simulink model "AUV_ControlsPreliminary"  (R2020b)
settings: Solver=ode23t  StartTime=0.0  StopTime=300  MaxStep=0.01  RelTol=1e-3  EnableMultiTasking=on
PreLoadFcn:
  | AUV_VehicleParameters;
  | Vehicle.Body.markeropacity = 0;
model workspace: external: MATLAB File AUV_DataFile_ORIG.m (data not in the file)
undefined symbols (not defined in the file or in its folder): Environment, Multibody, Newton, Raphson, smiData, X, x, Y, y, Z
libraries: sm_lib x3123, nesl_utility x51, sharedutil x8, pid_lib x6, AUVCustomPrimitives_Lib x4, shared6dof x1, aerolibasang x1, aerolibadyn x1, SignalEditorBlockLib x1
(part 4 of 62)

== system AUV_ControlsPreliminary/AUV/Muiltibody/World/Sea Floor ==
  T1 : sm_lib/Frames and Transforms/Rigid Transform  TranslationMethod=Cartesian  TranslationStandardOffset=0  TranslationLengthUnit=m  TranslationStandardAxis=+Z  TranslationCartesianOffset=[-Environment.seafloortileside 0 Environment.seafloordepth]  TranslationROffset=0  TranslationROffsetUnits=m  TranslationZOffset=0  TranslationZOffsetUnits=m  TranslationThetaOffset=0  TranslationThetaOffsetUnits=deg  RotationMethod=None  RotationAngleUnits=deg  RotationStandardAxis=+Z  RotationAngle=0.0  RotationArbitraryAxis=[0 0 1]  FollAlignAxisA=+X  BaseAlignAxisA=+Y  FollAlignAxisB=+Y  BaseAlignAxisB=+Z  RotationSequenceAxes=FollowerAxes  RotationSequence=XYX  RotationSequenceAngles=[0 0 0]  RotationSequenceAnglesUnits=deg  RotationMatrix=[1 0 0; 0 1 0; 0 0 1]
  Tiled Grid : Subsystem  mask(Tiled Grid){side=Environment.seafloortileside, thick=0.004, color1=[0 0.8 0.4], color2=[0 0.6 0.8], opacity=Environment.seaflooropacity}
      mask prompts: side "Tile Side (m) :"; thick "Tile Thickness (m) :"; color1 "First Color [RGB] :"; color2 "Second Color [RGB] :"; opacity "Tile Opacity (0...1) :"
      mask help: This block creates a tiled grid composed of square tiles.
  W : PMIOPort  Side=Left
  connections:
  W/RConn1 -- T1/LConn1
  T1/RConn1 -- Tiled Grid/LConn1

== system AUV_ControlsPreliminary/AUV/Singlebody/AUV Mechanics/DCMbe to R ==
  DCMbe : Inport
  Transpose : Math  Operator=transpose  SaturateOnIntegerOverflow=on
  R : Outport
  wires:
  Transpose/1 -> R/1
  DCMbe/1 -> Transpose/1

== system AUV_ControlsPreliminary/AUV/Singlebody/AUV Mechanics/Incidence Angles ==
  Vb : Inport
  "Incidence, Sideslip & Speed" : Subsystem
      mask Display:
      | port_label('input',1,'V_b','texmode','on');
      | port_label('output',1,'\alpha','texmode','on');
      | port_label('output',2,'\beta','texmode','on');
      | port_label('output',3,'V','texmode','on');
  alpha : Outport  Unit=rad
  beta : Outport  Port=2  Unit=rad
  V : Outport  Port=3  Unit=m/s
  wires:
  Vb/1 -> "Incidence, Sideslip & Speed"/1(Vb)
  "Incidence, Sideslip & Speed"/1(Alpha) -> alpha/1
  "Incidence, Sideslip & Speed"/3(V) -> V/1
  "Incidence, Sideslip & Speed"/2(Beta) -> beta/1

== system AUV_ControlsPreliminary/AUV/Singlebody/Hydro Forces & Moments/Added Mass Forces ==
  note: NOTE:
      | All added mass forces are already calculated with respect to the vehicle CoM
  AMFxyz : Inport
  AMMxyz : Inport  Port=2
  AMCFxyz : Inport  Port=3
  AMCMxyz : Inport  Port=4
  Sum : Sum  Inputs=|++
  Sum1 : Sum  Inputs=|++
  Fxyz : Outport
  Mxyz : Outport  Port=2
  wires:
  AMFxyz/1 -> Sum/1
  Sum/1 -> Fxyz/1
  AMCFxyz/1 -> Sum/2
  AMMxyz/1 -> Sum1/1
  Sum1/1 -> Mxyz/1
  AMCMxyz/1 -> Sum1/2

== system AUV_ControlsPreliminary/AUV/Singlebody/Hydro Forces & Moments/Hydrostatic Forces ==
  note: NOTE:
      | Both, the gravitaional force and the buoyancy force need to be transformed from inertial frame coordinates to body frame coordinates.
      | Additionally, the buoyancy force needs to be translated from the CoB to the CoM and we need to account for the corresponding moment.
  DCM : Inport
  Bz : Inport  Port=2
  Wz : Inport  Port=3
  CoB Moment Arm : Constant  Value=Vehicle.Body.Full.BArm
  Fb x (CoM-CoB) : sharedutil/3x3 Cross Product  aMode=aMode
      settings: SourceProductBaseCode=AE,PW,MT,UV,VE,VP
  Inertial to Body Buoyancy : Product  Multiplication=Matrix(*)
  Inertial to Body Weight : Product  Multiplication=Matrix(*)
  Reshape : Reshape  OutputDimensionality=Column vector (2-D)
  Sum : Sum  Inputs=++|
  Vector Concatenate : Concatenate  NumInputs=3
  Vector Concatenate1 : Concatenate  NumInputs=3
  zeroB : Constant  Value=0
  zeroW : Constant  Value=0
  Fxyz : Outport
  Mxyz : Outport  Port=2
  wires:
  Vector Concatenate1/1 -> Inertial to Body Weight/2
  DCM/1 -> Inertial to Body Weight/1, Inertial to Body Buoyancy/1
  Sum/1 -> Fxyz/1
  Inertial to Body Buoyancy/1 -> Sum/1, Fb x (CoM-CoB)/1  "Fb"
  zeroW/1 -> Vector Concatenate1/2, Vector Concatenate1/1
  Vector Concatenate/1 -> Inertial to Body Buoyancy/2
  zeroB/1 -> Vector Concatenate/2, Vector Concatenate/1
  Inertial to Body Weight/1 -> Sum/2  "Fg"
  Bz/1 -> Vector Concatenate/3
  Wz/1 -> Vector Concatenate1/3
  CoB Moment Arm/1 -> Reshape/1
  Fb x (CoM-CoB)/1 -> Mxyz/1
  Reshape/1 -> Fb x (CoM-CoB)/2

== system AUV_ControlsPreliminary/AUV/Singlebody/Hydro Forces & Moments/Lift and Drag Forces ==
  note: NOTE:
      | All lift and drag forces are already calculated with respect to the vehicle CoM
  LDFxyz : Inport
  LDMxyz : Inport  Port=2
  Fxyz : Outport
  Mxyz : Outport  Port=2
  wires:
  LDMxyz/1 -> Mxyz/1
  LDFxyz/1 -> Fxyz/1

== system AUV_ControlsPreliminary/AUV/Singlebody/Propellers & Thrusters/Horizontal Tunnel Thrusters ==
  note: NOTE:
      | Horizontal tunnel thruster vectors actuate in the +Y direction of the body frame
  BHTf : Inport
  SHTf : Inport  Port=2
  BHT Moment Arm wrt to CoM : Constant  Value=[Vehicle.Thruster.BHarmX,0,Vehicle.Thruster.BHarmZ]
  Fbht x (CoM-BHT) : sharedutil/3x3 Cross Product  aMode=aMode
      settings: SourceProductBaseCode=AE,PW,MT,UV,VE,VP
  Fsht x (CoM-SHT) : sharedutil/3x3 Cross Product  aMode=aMode
      settings: SourceProductBaseCode=AE,PW,MT,UV,VE,VP
  Reshape : Reshape  OutputDimensionality=Column vector (2-D)
  Reshape1 : Reshape  OutputDimensionality=Column vector (2-D)
  SHT Moment Arm wrt CoM : Constant  Value=[Vehicle.Thruster.SHarmX,0,Vehicle.Thruster.SHarmZ]
  Sum : Sum  Inputs=|++
  Sum1 : Sum  Inputs=|++
  Vector Concatenate : Concatenate  NumInputs=3
  Vector Concatenate1 : Concatenate  NumInputs=3
  zeroBHTf : Constant  Value=0
  zeroSHTf : Constant  Value=0
  Fxyz : Outport
  Mxyz : Outport  Port=2
  wires:
  zeroSHTf/1 -> Vector Concatenate1/3, Vector Concatenate1/1
  zeroBHTf/1 -> Vector Concatenate/3, Vector Concatenate/1
  Vector Concatenate/1 -> Fbht x (CoM-BHT)/1, Sum/1
  Vector Concatenate1/1 -> Fsht x (CoM-SHT)/1, Sum/2
  Sum/1 -> Fxyz/1
  BHT Moment Arm wrt to CoM/1 -> Reshape/1
  Reshape/1 -> Fbht x (CoM-BHT)/2
  SHT Moment Arm wrt CoM/1 -> Reshape1/1
  Sum1/1 -> Mxyz/1
  Fbht x (CoM-BHT)/1 -> Sum1/1
  Fsht x (CoM-SHT)/1 -> Sum1/2
  Reshape1/1 -> Fsht x (CoM-SHT)/2
  BHTf/1 -> Vector Concatenate/2
  SHTf/1 -> Vector Concatenate1/2

== system AUV_ControlsPreliminary/AUV/Singlebody/Propellers & Thrusters/Main Propellers ==
  note: NOTE:
      | Main propellers thrust vectors actuate in the +X direction of the body frame
  SPf : Inport
  PPf : Inport  Port=2
  Fpp x (CoM-PP) : sharedutil/3x3 Cross Product  aMode=aMode
      settings: SourceProductBaseCode=AE,PW,MT,UV,VE,VP
  Fsp x (CoM-SP) : sharedutil/3x3 Cross Product  aMode=aMode
      settings: SourceProductBaseCode=AE,PW,MT,UV,VE,VP
  PP Moment Arm wrt to CoM : Constant  Value=[0,Vehicle.Prop.PParmY,Vehicle.Prop.PParmZ]
  Reshape : Reshape  OutputDimensionality=Column vector (2-D)
  Reshape1 : Reshape  OutputDimensionality=Column vector (2-D)
  SP Moment Arm wrt to CoM : Constant  Value=[0,Vehicle.Prop.SParmY,Vehicle.Prop.SParmZ]
  Sum : Sum  Inputs=|++
  Sum1 : Sum  Inputs=|++
  Vector Concatenate : Concatenate  NumInputs=3
  Vector Concatenate1 : Concatenate  NumInputs=3
  zeroPPf : Constant  Value=0
  zeroSPf : Constant  Value=0
  Fxyz : Outport
  Mxyz : Outport  Port=2
  wires:
  PPf/1 -> Vector Concatenate1/1
  zeroSPf/1 -> Vector Concatenate/2, Vector Concatenate/3
  zeroPPf/1 -> Vector Concatenate1/2, Vector Concatenate1/3
  Vector Concatenate/1 -> Fsp x (CoM-SP)/1, Sum/1
  Vector Concatenate1/1 -> Fpp x (CoM-PP)/1, Sum/2
  SPf/1 -> Vector Concatenate/1
  Sum/1 -> Fxyz/1
  SP Moment Arm wrt to CoM/1 -> Reshape/1
  Reshape/1 -> Fsp x (CoM-SP)/2
  PP Moment Arm wrt to CoM/1 -> Reshape1/1
  Sum1/1 -> Mxyz/1
  Fsp x (CoM-SP)/1 -> Sum1/1
  Fpp x (CoM-PP)/1 -> Sum1/2
  Reshape1/1 -> Fpp x (CoM-PP)/2

== system AUV_ControlsPreliminary/AUV/Singlebody/Propellers & Thrusters/Vertical Tunnel Thrusters ==
  note: NOTE:
      | Vertical tunnel thruster vectors actuate in the +Z direction of the body frame
  BVTf : Inport
  SVTf : Inport  Port=2
  BVT Moment Arm wrt to CoM : Constant  Value=[Vehicle.Thruster.BVarmX,0,0]
  Fbvt x (CoM-BVT) : sharedutil/3x3 Cross Product  aMode=aMode
      settings: SourceProductBaseCode=AE,PW,MT,UV,VE,VP
  Fsvt x (CoM-SVT) : sharedutil/3x3 Cross Product  aMode=aMode
      settings: SourceProductBaseCode=AE,PW,MT,UV,VE,VP
  Reshape : Reshape  OutputDimensionality=Column vector (2-D)
  Reshape1 : Reshape  OutputDimensionality=Column vector (2-D)
  SVT Moment Arm wrt CoM : Constant  Value=[Vehicle.Thruster.SVarmX,0,0]
  Sum : Sum  Inputs=|++
  Sum1 : Sum  Inputs=|++
  Vector Concatenate : Concatenate  NumInputs=3
  Vector Concatenate1 : Concatenate  NumInputs=3
  zeroBVTf : Constant  Value=0
  zeroSVTf : Constant  Value=0
  Fxyz : Outport
  Mxyz : Outport  Port=2
  wires:
  Reshape1/1 -> Fsvt x (CoM-SVT)/2
  Fsvt x (CoM-SVT)/1 -> Sum1/2
  Fbvt x (CoM-BVT)/1 -> Sum1/1
  Sum1/1 -> Mxyz/1
  SVT Moment Arm wrt CoM/1 -> Reshape1/1
  Reshape/1 -> Fbvt x (CoM-BVT)/2
  BVT Moment Arm wrt to CoM/1 -> Reshape/1
  Sum/1 -> Fxyz/1
  Vector Concatenate1/1 -> Sum/2, Fsvt x (CoM-SVT)/1
  Vector Concatenate/1 -> Sum/1, Fbvt x (CoM-BVT)/1
  BVTf/1 -> Vector Concatenate/3
  zeroBVTf/1 -> Vector Concatenate/2, Vector Concatenate/1
  zeroSVTf/1 -> Vector Concatenate1/2, Vector Concatenate1/1
  SVTf/1 -> Vector Concatenate1/3

== system AUV_ControlsPreliminary/Dive Controls/Thrust Controls/Depth and Pitch Control/Main Propellers Thrust Offset Compensation ==
  PPf : Inport
  SPf : Inport  Port=2
  Bow Vertical Thruster Moment Arm : Constant  Value=-Vehicle.Thruster.BVarmX
  Main Propellers Moment Arm : Constant  Value=-Vehicle.Prop.SParmZ
  Product : Product
  Product1 : Product
  Product2 : Product  Inputs=*/
  Stern Vertical Thruster Moment Arm : Constant  Value=Vehicle.Thruster.SVarmX
  Sum : Sum  Inputs=|++
  Sum1 : Sum  Inputs=|++
  VTf : Outport
  wires:
  Product1/1 -> Sum/1
  Product/1 -> Sum/2
  SPf/1 -> Product/1
  PPf/1 -> Product1/1
  Main Propellers Moment Arm/1 -> Product1/2, Product/2
  Bow Vertical Thruster Moment Arm/1 -> Sum1/1
  Stern Vertical Thruster Moment Arm/1 -> Sum1/2
  Sum/1 -> Product2/1
  Sum1/1 -> Product2/2
  Product2/1 -> VTf/1

== system AUV_ControlsPreliminary/Dive Controls/Thrust Controls/Heading and Yaw Control/psidot ==
  pqr : Inport
  phithetapsi : Inport  Port=2
  Mux1 : Mux  Inputs=[3 3 3]
  psidot : Fcn  Expr=(u[2]*u[4]+u[3]*u[7])/u[8]
  sincos : Trigonometry  Operator=sincos
  psid : Outport  Unit=rad/s  InitialOutput=0  VectorParamsAs1DForOutWhenUnconnected=off
  wires:
  sincos/2 -> Mux1/3
  sincos/1 -> Mux1/2
  phithetapsi/1 -> sincos/1
  pqr/1 -> Mux1/1
  Mux1/1 -> psidot/1
  psidot/1 -> psid/1

== system AUV_ControlsPreliminary/Dive Controls/Thrust Controls/Heading and Yaw Control/side slip compensation ==
  note: NOTE: Lateral force offset is distributed based of the horizontal thrusters moment arms to make the net torque contribution zero
  v : Inport
  BowHTForce : Gain  Gain=Vehicle.Thruster.SHarmX/(-Vehicle.Thruster.BHarmX+Vehicle.Thruster.SHarmX)
  Gain1 : Gain  Gain=-1
  PIv : pid_lib/PID Controller  Controller=PI  Form=Parallel  TimeDomain=Continuous-time  UseExternalTs=off  SampleTime=-1  IntegratorMethod=Forward Euler  FilterMethod=Forward Euler  ControllerParametersSource=internal  P=10  I=0.01  D=0  UseFilter=on  N=100  TunerSelectOption=Transfer Function Based (PID Tuner App)  InitialConditionSource=internal  InitialConditionForIntegrator=0  InitialConditionForFilter=0  DifferentiatorICPrevScaledInput=0  ExternalReset=none  TrackingMode=off  Kt=1  LimitOutput=off  SatLimitsSource=internal  UpperSaturationLimit=inf  LowerSaturationLimit=-inf  LinearizeAsGain=on  AntiWindupMode=none  Kb=1  POutMin=[]  POutMax=[]  IOutMin=[]  IOutMax=[]  DOutMin=[]  DOutMax=[]  NOutMin=[]  NOutMax=[]  SumOutMin=[]  SumOutMax=[]  SaturationOutMin=[]  SaturationOutMax=[]  PParamMin=[]  PParamMax=[]  IParamMin=[]  IParamMax=[]  DParamMin=[]  DParamMax=[]  NParamMin=[]  NParamMax=[]  KbParamMin=[]  KbParamMax=[]  KtParamMin=[]  KtParamMax=[]  KbOutMin=[]  KbOutMax=[]  KtOutMin=[]  KtOutMax=[]  IntegratorOutMin=[]  IntegratorOutMax=[]  FilterOutMin=[]  FilterOutMax=[]  SumI1OutMin=[]  SumI1OutMax=[]  SumI2OutMin=[]  SumI2OutMax=[]  SumI3OutMin=[]  SumI3OutMax=[]  SumI4OutMin=[]  SumI4OutMax=[]  SumDOutMin=[]  SumDOutMax=[]  DifferentiatorOutMin=[]  DifferentiatorOutMax=[]  FilterDiffOutCoefMin=[]  FilterDiffOutCoefMax=[]  ReciprocalOutMin=[]  ReciprocalOutMax=[]  SumDenOutMin=[]  SumDenOutMax=[]  SumNumOutMin=[]  SumNumOutMax=[]  DivideOutMin=[]  DivideOutMax=[]  UdiffTsProdOutMin=[]  UdiffTsProdOutMax=[]  NTsProdOutMin=[]  NTsProdOutMax=[]  UintegralTsProdOutMin=[]  UintegralTsProdOutMax=[]  UngainTsProdOutMin=[]  UngainTsProdOutMax=[]  IntegratorContinuousStateAttributes=''  IntegratorStateMustResolveToSignalObject=off  IntegratorRTWStateStorageClass=Auto  FilterContinuousStateAttributes=''  FilterStateMustResolveToSignalObject=off  FilterRTWStateStorageClass=Auto  ParallelPVariant=InternalParameters  IdealPVariant=Disabled  IVariant=InternalParameters  DVariant=Disabled  IntegratorVariant=Continuous  SatVariant=Disabled  AWVariant=Passthrough  PCopyVariant=Disabled  TRVariant=Disabled  FdbkBlocksVariant=Forward  IdealPFdbkVariant=Disabled  SatFdbkVariant=Disabled  DerivativeFilterVariant=Disabled  NVariant=Disabled  NCopyVariant=Disabled_SignalSpec  FilterICVariant=Disabled  IntegratorICVariant=InternalICs  ExternalResetVariant=Disabled  TRSumVariant=Passthrough  SumFdbkVariant=Disabled  SumVariant=Sum_PI  TsampFilterVariant=InternalTs  TsampNgainVariant=Passthrough  TsampIntegralVariant=Passthrough  ExternalSaturationOutDataTypeStr=Inherit: Same as second input
  SternHTForce : Gain  Gain=-Vehicle.Thruster.BHarmX/(-Vehicle.Thruster.BHarmX+Vehicle.Thruster.SHarmX)
  BHTf : Outport
  SHTf : Outport  Port=2
  wires:
  Gain1/1 -> PIv/1
  SternHTForce/1 -> SHTf/1
  PIv/1 -> BowHTForce/1, SternHTForce/1
  v/1 -> Gain1/1
  BowHTForce/1 -> BHTf/1

== system AUV_ControlsPreliminary/Hydrostatic & Hydrodynamic Effects/Added Mass Forces/Added Mass/LPfilter ==
  note: NOTE:
      | Using low pass filters with
      | 1 milisecond time constant
      | to break the algebraic loop
  in : Inport
  Demux : Demux  Outputs=6
  LPfilter{1..6} (6 alike) : TransferFcn  Denominator=[0.001 1]
  Mux : Mux  Inputs=6
  out : Outport
  wires:
  Demux/1 -> LPfilter1/1
  Demux/2 -> LPfilter2/1
  in/1 -> Demux/1
  Demux/6 -> LPfilter6/1
  Demux/5 -> LPfilter5/1
  Demux/4 -> LPfilter4/1
  Demux/3 -> LPfilter3/1
  LPfilter1/1 -> Mux/1
  LPfilter2/1 -> Mux/2
  LPfilter3/1 -> Mux/3
  LPfilter4/1 -> Mux/4
  LPfilter5/1 -> Mux/5
  LPfilter6/1 -> Mux/6
  Mux/1 -> out/1

== system AUV_ControlsPreliminary/Hydrostatic & Hydrodynamic Effects/Added Mass Forces/Coriolis/Ca(V) ==
  note: $a_1 = m_{11}u \\ a_2 = m_{22}v+m_{26}r\\ a_3 = m_{33}w+m_{35}q\\ b_1 = m_{44}p\\ b_2 = m_{53}w+m_{55}q\\ b_3 = m_{62}v+m_{66}r$
  a1 : Inport
  a2 : Inport  Port=2
  a3 : Inport  Port=3
  b1 : Inport  Port=4
  b2 : Inport  Port=5
  b3 : Inport  Port=6
  Matrix Concatenate : Concatenate  NumInputs=6  Mode=Multidimensional array
  row1 : Subsystem
  row2 : Subsystem
  row3 : Subsystem
  row4 : Subsystem
  row5 : Subsystem
  row6 : Subsystem
  Ca(V) : Outport
  wires:
  a2/1 -> row1/1(a2), row3/2(a2), row6/2(a2), row4/1(a2)
  b3/1 -> row5/4(b3), row4/4(b3)
  b2/1 -> row4/3(b2), row6/4(b2)
  a1/1 -> row6/1(a1), row5/1(a1), row3/1(a1), row2/1(a1)
  row1/1(row1) -> Matrix Concatenate/1
  row2/1(row2) -> Matrix Concatenate/2
  row3/1(row3) -> Matrix Concatenate/3
  a3/1 -> row5/2(a3), row4/2(a3), row1/2(a3), row2/2(a3)
  row4/1(row4) -> Matrix Concatenate/4
  b1/1 -> row5/3(b1), row6/3(b1)
  row6/1(row6) -> Matrix Concatenate/6
  row5/1(row5) -> Matrix Concatenate/5
  Matrix Concatenate/1 -> Ca(V)/1

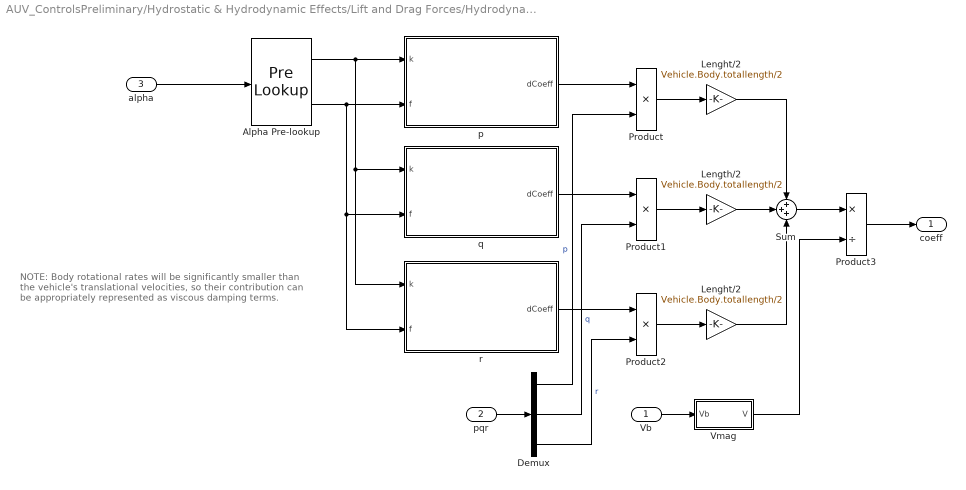
== system AUV_ControlsPreliminary/Hydrostatic & Hydrodynamic Effects/Lift and Drag Forces/Hydrodynamic Coefficients/Body Rate Damping ==
  note: NOTE:
      | Body rotational rates will be significantly smaller
      | than the vehicle's translational velocities, so their
      | contribution can be appropriately represented as
      | viscous damping terms.
  Vb : Inport
  pqr : Inport  Port=2
  alpha : Inport  Port=3  Unit=deg
  Alpha Pre-lookup : PreLookup  BreakpointsData=Vehicle.IncRange.alpha_vec_damp  ExtrapMethod=Linear
  Demux : Demux  Outputs=3
  "Lenght/2 " : Gain  Gain=Vehicle.Body.totallength/2
  "Lenght/2  " : Gain  Gain=Vehicle.Body.totallength/2
  Length/2 : Gain  Gain=Vehicle.Body.totallength/2
  Product : Product
  Product1 : Product
  Product2 : Product
  Product3 : Product  Inputs=*/
  Sum : Sum  Inputs=+++
  Vmag : Subsystem
  p : Subsystem
  q : Subsystem
  r : Subsystem
  coeff : Outport
  wires:
  pqr/1 -> Demux/1
  alpha/1 -> Alpha Pre-lookup/1
  Alpha Pre-lookup/1 -> q/1(k), r/1(k), p/1(k)
  Alpha Pre-lookup/2 -> r/2(f), q/2(f), p/2(f)
  p/1(dCoeff) -> Product/1
  q/1(dCoeff) -> Product1/1
  r/1(dCoeff) -> Product2/1
  Demux/3 -> Product2/2  "r"
  Demux/2 -> Product1/2  "q"
  Demux/1 -> Product/2  "p"
  Product1/1 -> Length/2/1
  Product/1 -> "Lenght/2  "/1
  Product2/1 -> "Lenght/2 "/1
  Sum/1 -> Product3/1
  Vb/1 -> Vmag/1(Vb)
  Vmag/1(V) -> Product3/2
  Product3/1 -> coeff/1
  "Lenght/2  "/1 -> Sum/1
  Length/2/1 -> Sum/2
  "Lenght/2 "/1 -> Sum/3

== system AUV_ControlsPreliminary/Hydrostatic & Hydrodynamic Effects/Lift and Drag Forces/Hydrodynamic Coefficients/Drag and Lift Coefficients ==
  alpha : Inport  Unit=deg
  beta : Inport  Port=2  Unit=deg
  Alpha Pre-lookup : PreLookup  BreakpointsData=Vehicle.IncRange.alpha_vec  ExtrapMethod=Linear
  Beta Pre-lookup : PreLookup  BreakpointsData=Vehicle.IncRange.beta_vec  ExtrapMethod=Linear
  CMK : Interpolation_n-D  Table=Vehicle.Coeff.CMK'  InternalRulePriority=Speed
  CMM : Interpolation_n-D  Table=Vehicle.Coeff.CMM'  InternalRulePriority=Speed
  CMN : Interpolation_n-D  Table=Vehicle.Coeff.CMN'  InternalRulePriority=Speed
  CX : Interpolation_n-D  Table=Vehicle.Coeff.CX'  InternalRulePriority=Speed
  CY : Interpolation_n-D  Table=Vehicle.Coeff.CY'  InternalRulePriority=Speed
  CZ : Interpolation_n-D  Table=Vehicle.Coeff.CZ'  InternalRulePriority=Speed
  Gain : Gain  Gain=0.001
  Mux : Mux  Inputs=6
  coeff : Outport
  wires:
  alpha/1 -> Alpha Pre-lookup/1
  beta/1 -> Beta Pre-lookup/1
  Mux/1 -> coeff/1
  Alpha Pre-lookup/1 -> CMN/1, CMM/1, CMK/1, CZ/1, CY/1, CX/1
  Alpha Pre-lookup/2 -> CMK/2, CMM/2, CMN/2, CZ/2, CY/2, CX/2
  CX/1 -> Mux/1
  Beta Pre-lookup/1 -> CMM/3, CMN/3, CMK/3, CZ/3, CY/3, CX/3
  Beta Pre-lookup/2 -> CMM/4, CMN/4, CMK/4, CZ/4, CY/4, CX/4
  CY/1 -> Mux/2
  CZ/1 -> Mux/3
  CMK/1 -> Gain/1
  CMM/1 -> Mux/5
  CMN/1 -> Mux/6
  Gain/1 -> Mux/4

== system AUV_ControlsPreliminary/AUV/Muiltibody/AUV Mechanics/AUVBody/BowHorThrusterTunnel ==
  Altimeter : Subsystem
      mask Display: image('Altimeter.png')
  BowHorThrusterMount : Subsystem
      mask Display: image('ThrusterMount.png')
  Bow_Horizontal_Thruster_Tunnel : Subsystem
      mask Display: image('HorizontalTunnelBow.png')
  Depth_Sensor : Subsystem
      mask Display: image('Depth.png')
  ReferenceFrame : sm_lib/Frames and Transforms/Reference Frame
  T1 : sm_lib/Frames and Transforms/Rigid Transform  TranslationMethod=Cartesian  TranslationStandardOffset=0  TranslationLengthUnit=m  TranslationStandardAxis=+Z  TranslationCartesianOffset=smiData.RigidTransform(24).translation  TranslationROffset=0  TranslationROffsetUnits=m  TranslationZOffset=0  TranslationZOffsetUnits=m  TranslationThetaOffset=0  TranslationThetaOffsetUnits=deg  RotationMethod=ArbitraryAxis  RotationAngleUnits=rad  RotationStandardAxis=+Z  RotationAngle=smiData.RigidTransform(24).angle  RotationArbitraryAxis=smiData.RigidTransform(24).axis  FollAlignAxisA=+X  BaseAlignAxisA=+Y  FollAlignAxisB=+Y  BaseAlignAxisB=+Z  RotationSequenceAxes=FollowerAxes  RotationSequence=XYX  RotationSequenceAngles=[0 0 0]  RotationSequenceAnglesUnits=deg  RotationMatrix=[1 0 0; 0 1 0; 0 0 1]
  T2 : sm_lib/Frames and Transforms/Rigid Transform  TranslationMethod=Cartesian  TranslationStandardOffset=0  TranslationLengthUnit=m  TranslationStandardAxis=+Z  TranslationCartesianOffset=smiData.RigidTransform(25).translation  TranslationROffset=0  TranslationROffsetUnits=m  TranslationZOffset=0  TranslationZOffsetUnits=m  TranslationThetaOffset=0  TranslationThetaOffsetUnits=deg  RotationMethod=ArbitraryAxis  RotationAngleUnits=rad  RotationStandardAxis=+Z  RotationAngle=smiData.RigidTransform(25).angle  RotationArbitraryAxis=smiData.RigidTransform(25).axis  FollAlignAxisA=+X  BaseAlignAxisA=+Y  FollAlignAxisB=+Y  BaseAlignAxisB=+Z  RotationSequenceAxes=FollowerAxes  RotationSequence=XYX  RotationSequenceAngles=[0 0 0]  RotationSequenceAnglesUnits=deg  RotationMatrix=[1 0 0; 0 1 0; 0 0 1]
  T3 : sm_lib/Frames and Transforms/Rigid Transform  TranslationMethod=Cartesian  TranslationStandardOffset=0  TranslationLengthUnit=m  TranslationStandardAxis=+Z  TranslationCartesianOffset=smiData.RigidTransform(26).translation  TranslationROffset=0  TranslationROffsetUnits=m  TranslationZOffset=0  TranslationZOffsetUnits=m  TranslationThetaOffset=0  TranslationThetaOffsetUnits=deg  RotationMethod=ArbitraryAxis  RotationAngleUnits=rad  RotationStandardAxis=+Z  RotationAngle=smiData.RigidTransform(26).angle  RotationArbitraryAxis=smiData.RigidTransform(26).axis  FollAlignAxisA=+X  BaseAlignAxisA=+Y  FollAlignAxisB=+Y  BaseAlignAxisB=+Z  RotationSequenceAxes=FollowerAxes  RotationSequence=XYX  RotationSequenceAngles=[0 0 0]  RotationSequenceAnglesUnits=deg  RotationMatrix=[1 0 0; 0 1 0; 0 0 1]
  T4 : sm_lib/Frames and Transforms/Rigid Transform  TranslationMethod=Cartesian  TranslationStandardOffset=0  TranslationLengthUnit=m  TranslationStandardAxis=+Z  TranslationCartesianOffset=smiData.RigidTransform(27).translation  TranslationROffset=0  TranslationROffsetUnits=m  TranslationZOffset=0  TranslationZOffsetUnits=m  TranslationThetaOffset=0  TranslationThetaOffsetUnits=deg  RotationMethod=ArbitraryAxis  RotationAngleUnits=rad  RotationStandardAxis=+Z  RotationAngle=smiData.RigidTransform(27).angle  RotationArbitraryAxis=smiData.RigidTransform(27).axis  FollAlignAxisA=+X  BaseAlignAxisA=+Y  FollAlignAxisB=+Y  BaseAlignAxisB=+Z  RotationSequenceAxes=FollowerAxes  RotationSequence=XYX  RotationSequenceAngles=[0 0 0]  RotationSequenceAnglesUnits=deg  RotationMatrix=[1 0 0; 0 1 0; 0 0 1]
  T5 : sm_lib/Frames and Transforms/Rigid Transform  TranslationMethod=Cartesian  TranslationStandardOffset=0  TranslationLengthUnit=m  TranslationStandardAxis=+Z  TranslationCartesianOffset=smiData.RigidTransform(9).translation  TranslationROffset=0  TranslationROffsetUnits=m  TranslationZOffset=0  TranslationZOffsetUnits=m  TranslationThetaOffset=0  TranslationThetaOffsetUnits=deg  RotationMethod=ArbitraryAxis  RotationAngleUnits=rad  RotationStandardAxis=+Z  RotationAngle=smiData.RigidTransform(9).angle  RotationArbitraryAxis=smiData.RigidTransform(9).axis  FollAlignAxisA=+X  BaseAlignAxisA=+Y  FollAlignAxisB=+Y  BaseAlignAxisB=+Z  RotationSequenceAxes=FollowerAxes  RotationSequence=XYX  RotationSequenceAngles=[0 0 0]  RotationSequenceAnglesUnits=deg  RotationMatrix=[1 0 0; 0 1 0; 0 0 1]
  F : PMIOPort  Side=Left
  BHT : PMIOPort  Port=2  Side=Right
  connections:
  T4/LConn1 -- F/RConn1 -- T5/LConn1
  T1/LConn1 -- T2/LConn1 -- ReferenceFrame/RConn1 -- T3/LConn1 -- T4/RConn1 -- BowHorThrusterMount/RConn1
  Bow_Horizontal_Thruster_Tunnel/LConn1 -- T3/RConn1
  Altimeter/LConn1 -- T2/RConn1
  Depth_Sensor/LConn1 -- T1/RConn1
  BHT/RConn1 -- T5/RConn1

== system AUV_ControlsPreliminary/AUV/Muiltibody/AUV Mechanics/AUVBody/BowHullCap ==
  Bow_Hull_Cap : Subsystem
      mask Display: image('BowHullCap.png')
  Bow_Sensors : Subsystem
      mask Display: image('BowSensors.png')
  Front_Camera : Subsystem
      mask Display: image('FCamera.png')
  ReferenceFrame : sm_lib/Frames and Transforms/Reference Frame
  T1 : sm_lib/Frames and Transforms/Rigid Transform  TranslationMethod=Cartesian  TranslationStandardOffset=0  TranslationLengthUnit=m  TranslationStandardAxis=+Z  TranslationCartesianOffset=smiData.RigidTransform(28).translation  TranslationROffset=0  TranslationROffsetUnits=m  TranslationZOffset=0  TranslationZOffsetUnits=m  TranslationThetaOffset=0  TranslationThetaOffsetUnits=deg  RotationMethod=ArbitraryAxis  RotationAngleUnits=rad  RotationStandardAxis=+Z  RotationAngle=smiData.RigidTransform(28).angle  RotationArbitraryAxis=smiData.RigidTransform(28).axis  FollAlignAxisA=+X  BaseAlignAxisA=+Y  FollAlignAxisB=+Y  BaseAlignAxisB=+Z  RotationSequenceAxes=FollowerAxes  RotationSequence=XYX  RotationSequenceAngles=[0 0 0]  RotationSequenceAnglesUnits=deg  RotationMatrix=[1 0 0; 0 1 0; 0 0 1]
  T2 : sm_lib/Frames and Transforms/Rigid Transform  TranslationMethod=Cartesian  TranslationStandardOffset=0  TranslationLengthUnit=m  TranslationStandardAxis=+Z  TranslationCartesianOffset=smiData.RigidTransform(29).translation  TranslationROffset=0  TranslationROffsetUnits=m  TranslationZOffset=0  TranslationZOffsetUnits=m  TranslationThetaOffset=0  TranslationThetaOffsetUnits=deg  RotationMethod=ArbitraryAxis  RotationAngleUnits=rad  RotationStandardAxis=+Z  RotationAngle=smiData.RigidTransform(29).angle  RotationArbitraryAxis=smiData.RigidTransform(29).axis  FollAlignAxisA=+X  BaseAlignAxisA=+Y  FollAlignAxisB=+Y  BaseAlignAxisB=+Z  RotationSequenceAxes=FollowerAxes  RotationSequence=XYX  RotationSequenceAngles=[0 0 0]  RotationSequenceAnglesUnits=deg  RotationMatrix=[1 0 0; 0 1 0; 0 0 1]
  T3 : sm_lib/Frames and Transforms/Rigid Transform  TranslationMethod=Cartesian  TranslationStandardOffset=0  TranslationLengthUnit=m  TranslationStandardAxis=+Z  TranslationCartesianOffset=smiData.RigidTransform(30).translation  TranslationROffset=0  TranslationROffsetUnits=m  TranslationZOffset=0  TranslationZOffsetUnits=m  TranslationThetaOffset=0  TranslationThetaOffsetUnits=deg  RotationMethod=ArbitraryAxis  RotationAngleUnits=rad  RotationStandardAxis=+Z  RotationAngle=smiData.RigidTransform(30).angle  RotationArbitraryAxis=smiData.RigidTransform(30).axis  FollAlignAxisA=+X  BaseAlignAxisA=+Y  FollAlignAxisB=+Y  BaseAlignAxisB=+Z  RotationSequenceAxes=FollowerAxes  RotationSequence=XYX  RotationSequenceAngles=[0 0 0]  RotationSequenceAnglesUnits=deg  RotationMatrix=[1 0 0; 0 1 0; 0 0 1]
  T4 : sm_lib/Frames and Transforms/Rigid Transform  TranslationMethod=StandardAxis  TranslationStandardOffset=-0.036  TranslationLengthUnit=m  TranslationStandardAxis=+Z  TranslationCartesianOffset=[0 0 0]  TranslationROffset=0  TranslationROffsetUnits=m  TranslationZOffset=0  TranslationZOffsetUnits=m  TranslationThetaOffset=0  TranslationThetaOffsetUnits=deg  RotationMethod=None  RotationAngleUnits=deg  RotationStandardAxis=+Z  RotationAngle=0.0  RotationArbitraryAxis=[0 0 1]  FollAlignAxisA=+X  BaseAlignAxisA=+Y  FollAlignAxisB=+Y  BaseAlignAxisB=+Z  RotationSequenceAxes=FollowerAxes  RotationSequence=XYX  RotationSequenceAngles=[0 0 0]  RotationSequenceAnglesUnits=deg  RotationMatrix=[1 0 0; 0 1 0; 0 0 1]
  Tip : PMIOPort  Side=Left
  F : PMIOPort  Port=2  Side=Left
  connections:
  Front_Camera/LConn1 -- T4/RConn1
  T3/LConn1 -- F/RConn1
  T2/LConn1 -- T3/RConn1 -- T4/LConn1 -- ReferenceFrame/RConn1 -- T1/LConn1
  Bow_Sensors/LConn1 -- T2/RConn1
  Bow_Hull_Cap/LConn1 -- T1/RConn1
  Tip/RConn1 -- Bow_Hull_Cap/RConn1

== system AUV_ControlsPreliminary/AUV/Muiltibody/AUV Mechanics/AUVBody/BowVerThrusterTunnel ==
  BowVerThrusterMount : Subsystem
      mask Display: image('ThrusterMount.png')
  Bow_Vertical_Thruster_Tunnel : Subsystem
      mask Display: image('VerticalTunnel.png')
  ReferenceFrame : sm_lib/Frames and Transforms/Reference Frame
  T1 : sm_lib/Frames and Transforms/Rigid Transform  TranslationMethod=Cartesian  TranslationStandardOffset=0  TranslationLengthUnit=m  TranslationStandardAxis=+Z  TranslationCartesianOffset=smiData.RigidTransform(39).translation  TranslationROffset=0  TranslationROffsetUnits=m  TranslationZOffset=0  TranslationZOffsetUnits=m  TranslationThetaOffset=0  TranslationThetaOffsetUnits=deg  RotationMethod=ArbitraryAxis  RotationAngleUnits=rad  RotationStandardAxis=+Z  RotationAngle=smiData.RigidTransform(39).angle  RotationArbitraryAxis=smiData.RigidTransform(39).axis  FollAlignAxisA=+X  BaseAlignAxisA=+Y  FollAlignAxisB=+Y  BaseAlignAxisB=+Z  RotationSequenceAxes=FollowerAxes  RotationSequence=XYX  RotationSequenceAngles=[0 0 0]  RotationSequenceAnglesUnits=deg  RotationMatrix=[1 0 0; 0 1 0; 0 0 1]
  T2 : sm_lib/Frames and Transforms/Rigid Transform  TranslationMethod=Cartesian  TranslationStandardOffset=0  TranslationLengthUnit=m  TranslationStandardAxis=+Z  TranslationCartesianOffset=smiData.RigidTransform(40).translation  TranslationROffset=0  TranslationROffsetUnits=m  TranslationZOffset=0  TranslationZOffsetUnits=m  TranslationThetaOffset=0  TranslationThetaOffsetUnits=deg  RotationMethod=ArbitraryAxis  RotationAngleUnits=rad  RotationStandardAxis=+Z  RotationAngle=smiData.RigidTransform(40).angle  RotationArbitraryAxis=smiData.RigidTransform(40).axis  FollAlignAxisA=+X  BaseAlignAxisA=+Y  FollAlignAxisB=+Y  BaseAlignAxisB=+Z  RotationSequenceAxes=FollowerAxes  RotationSequence=XYX  RotationSequenceAngles=[0 0 0]  RotationSequenceAnglesUnits=deg  RotationMatrix=[1 0 0; 0 1 0; 0 0 1]
  T3 : sm_lib/Frames and Transforms/Rigid Transform  TranslationMethod=Cartesian  TranslationStandardOffset=0  TranslationLengthUnit=m  TranslationStandardAxis=+Z  TranslationCartesianOffset=smiData.RigidTransform(3).translation  TranslationROffset=0  TranslationROffsetUnits=m  TranslationZOffset=0  TranslationZOffsetUnits=m  TranslationThetaOffset=0  TranslationThetaOffsetUnits=deg  RotationMethod=ArbitraryAxis  RotationAngleUnits=rad  RotationStandardAxis=+Z  RotationAngle=smiData.RigidTransform(3).angle  RotationArbitraryAxis=smiData.RigidTransform(3).axis  FollAlignAxisA=+X  BaseAlignAxisA=+Y  FollAlignAxisB=+Y  BaseAlignAxisB=+Z  RotationSequenceAxes=FollowerAxes  RotationSequence=XYX  RotationSequenceAngles=[0 0 0]  RotationSequenceAnglesUnits=deg  RotationMatrix=[1 0 0; 0 1 0; 0 0 1]
  F : PMIOPort  Side=Left
  BVT : PMIOPort  Port=2  Side=Right
  connections:
  T2/LConn1 -- F/RConn1 -- T3/LConn1
  ReferenceFrame/RConn1 -- T1/LConn1 -- T2/RConn1 -- BowVerThrusterMount/LConn1
  Bow_Vertical_Thruster_Tunnel/LConn1 -- T1/RConn1
  BVT/RConn1 -- T3/RConn1

== system AUV_ControlsPreliminary/AUV/Muiltibody/AUV Mechanics/AUVBody/MainHull ==
  BatteryPack : Subsystem
      settings: PortSchema="{\"entries\":[{\"content\":{\"sides\":[{\"content\":{\"connectorIds\":[]},\"type\":\"ConnectorPlacement.EquallySpacedRectSide\",\"uuid\":\"9b8fdd88-1c7e-48be-9cfb-0481a6997d70\"},{\"content\":{\"connectorIds\":[],\"side\":\"RIGHT\"},\"type\":\"ConnectorPlacement.EquallySpacedRectSide\",\"uuid\":\"09133262-ae09-4a08-942a-feb1f9e4bf66\"},{\"content\":{\"connectorIds\":[\"LConn1\"],\"side\":\"TOP\"},\"type\":\"ConnectorPlacement.EquallySpacedRectSide\",\"uuid\":\"b524eb7e-dd7a-431a-8842-4adf3b6cfedc\"}]},\"type\":\"ConnectorPlacement.EquallySpacedConnector\",\"uuid\":\"16ac0096-5732-49f8-94c0-648a6a453a34\"}],\"packageUris\":[\"http://schema.mathworks.com/mf0/Connector/19700101\"],\"version\":\"1.0\"}"
      mask Display: image('BatteryPack.png')
  BottomStrip : Subsystem
      settings: PortSchema="{\"entries\":[{\"content\":{\"sides\":[{\"content\":{\"connectorIds\":[]},\"type\":\"ConnectorPlacement.EquallySpacedRectSide\",\"uuid\":\"9b8fdd88-1c7e-48be-9cfb-0481a6997d70\"},{\"content\":{\"connectorIds\":[],\"side\":\"RIGHT\"},\"type\":\"ConnectorPlacement.EquallySpacedRectSide\",\"uuid\":\"09133262-ae09-4a08-942a-feb1f9e4bf66\"},{\"content\":{\"connectorIds\":[\"LConn1\"],\"side\":\"TOP\"},\"type\":\"ConnectorPlacement.EquallySpacedRectSide\",\"uuid\":\"b524eb7e-dd7a-431a-8842-4adf3b6cfedc\"}]},\"type\":\"ConnectorPlacement.EquallySpacedConnector\",\"uuid\":\"16ac0096-5732-49f8-94c0-648a6a453a34\"}],\"packageUris\":[\"http://schema.mathworks.com/mf0/Connector/19700101\"],\"version\":\"1.0\"}"
      mask Display: image('BottomStrip.png')
  Camera : Subsystem
      settings: PortSchema="{\"entries\":[{\"content\":{\"sides\":[{\"content\":{\"connectorIds\":[]},\"type\":\"ConnectorPlacement.EquallySpacedRectSide\",\"uuid\":\"9b8fdd88-1c7e-48be-9cfb-0481a6997d70\"},{\"content\":{\"connectorIds\":[],\"side\":\"RIGHT\"},\"type\":\"ConnectorPlacement.EquallySpacedRectSide\",\"uuid\":\"09133262-ae09-4a08-942a-feb1f9e4bf66\"},{\"content\":{\"connectorIds\":[\"LConn1\"],\"side\":\"TOP\"},\"type\":\"ConnectorPlacement.EquallySpacedRectSide\",\"uuid\":\"b524eb7e-dd7a-431a-8842-4adf3b6cfedc\"}]},\"type\":\"ConnectorPlacement.EquallySpacedConnector\",\"uuid\":\"16ac0096-5732-49f8-94c0-648a6a453a34\"}],\"packageUris\":[\"http://schema.mathworks.com/mf0/Connector/19700101\"],\"version\":\"1.0\"}"
      mask Display: image('Camera.png')
  DVL : Subsystem
      settings: PortSchema="{\"entries\":[{\"content\":{\"sides\":[{\"content\":{\"connectorIds\":[]},\"type\":\"ConnectorPlacement.EquallySpacedRectSide\",\"uuid\":\"9b8fdd88-1c7e-48be-9cfb-0481a6997d70\"},{\"content\":{\"connectorIds\":[],\"side\":\"RIGHT\"},\"type\":\"ConnectorPlacement.EquallySpacedRectSide\",\"uuid\":\"09133262-ae09-4a08-942a-feb1f9e4bf66\"},{\"content\":{\"connectorIds\":[\"LConn1\"],\"side\":\"TOP\"},\"type\":\"ConnectorPlacement.EquallySpacedRectSide\",\"uuid\":\"b524eb7e-dd7a-431a-8842-4adf3b6cfedc\"}]},\"type\":\"ConnectorPlacement.EquallySpacedConnector\",\"uuid\":\"16ac0096-5732-49f8-94c0-648a6a453a34\"}],\"packageUris\":[\"http://schema.mathworks.com/mf0/Connector/19700101\"],\"version\":\"1.0\"}"
      mask Display: image('DVL.png')
  ElectronicBoards : Subsystem
      settings: PortSchema="{\"entries\":[{\"content\":{\"sides\":[{\"content\":{\"connectorIds\":[\"LConn1\"]},\"type\":\"ConnectorPlacement.EquallySpacedRectSide\",\"uuid\":\"ee174d83-7ec9-4f78-977a-5ac618f84910\"},{\"content\":{\"connectorIds\":[],\"side\":\"RIGHT\"},\"type\":\"ConnectorPlacement.EquallySpacedRectSide\",\"uuid\":\"b1f8772f-a994-4bc2-984b-3dde78400d8f\"},{\"content\":{\"connectorIds\":[\"LConn2\"],\"side\":\"TOP\"},\"type\":\"ConnectorPlacement.EquallySpacedRectSide\",\"uuid\":\"f9256764-d20c-453c-9456-9dc5ed28a8dc\"}]},\"type\":\"ConnectorPlacement.EquallySpacedConnector\",\"uuid\":\"1072f53a-ce7b-4a5a-9466-cf066be5f153\"}],\"packageUris\":[\"http://schema.mathworks.com/mf0/Connector/19700101\"],\"version\":\"1.0\"}"
      mask Display: image('Electronics.png')
  Frame Alignment : Subsystem
  GPS : Subsystem
      settings: PortSchema="{\"entries\":[{\"content\":{\"sides\":[{\"content\":{\"connectorIds\":[]},\"type\":\"ConnectorPlacement.EquallySpacedRectSide\",\"uuid\":\"9b8fdd88-1c7e-48be-9cfb-0481a6997d70\"},{\"content\":{\"connectorIds\":[],\"side\":\"RIGHT\"},\"type\":\"ConnectorPlacement.EquallySpacedRectSide\",\"uuid\":\"09133262-ae09-4a08-942a-feb1f9e4bf66\"},{\"content\":{\"connectorIds\":[\"LConn1\"],\"side\":\"TOP\"},\"type\":\"ConnectorPlacement.EquallySpacedRectSide\",\"uuid\":\"b524eb7e-dd7a-431a-8842-4adf3b6cfedc\"}]},\"type\":\"ConnectorPlacement.EquallySpacedConnector\",\"uuid\":\"16ac0096-5732-49f8-94c0-648a6a453a34\"}],\"packageUris\":[\"http://schema.mathworks.com/mf0/Connector/19700101\"],\"version\":\"1.0\"}"
      mask Display: image('GPS.png')
  Main_Hull : Subsystem
      settings: PortSchema="{\"entries\":[{\"content\":{\"sides\":[{\"content\":{\"connectorIds\":[]},\"type\":\"ConnectorPlacement.EquallySpacedRectSide\",\"uuid\":\"9b8fdd88-1c7e-48be-9cfb-0481a6997d70\"},{\"content\":{\"connectorIds\":[],\"side\":\"RIGHT\"},\"type\":\"ConnectorPlacement.EquallySpacedRectSide\",\"uuid\":\"09133262-ae09-4a08-942a-feb1f9e4bf66\"},{\"content\":{\"connectorIds\":[\"LConn1\"],\"side\":\"TOP\"},\"type\":\"ConnectorPlacement.EquallySpacedRectSide\",\"uuid\":\"b524eb7e-dd7a-431a-8842-4adf3b6cfedc\"}]},\"type\":\"ConnectorPlacement.EquallySpacedConnector\",\"uuid\":\"16ac0096-5732-49f8-94c0-648a6a453a34\"}],\"packageUris\":[\"http://schema.mathworks.com/mf0/Connector/19700101\"],\"version\":\"1.0\"}"
      mask Display: image('Hull.png',[0,0.05,1,0.9])
  PortPropMotor : Subsystem
      mask Display: image('PropMotor.png',[0,0.05,1,0.9])
  ReferenceFrame : sm_lib/Frames and Transforms/Reference Frame
  Sonar1 : Subsystem
      settings: PortSchema="{\"entries\":[{\"content\":{\"sides\":[{\"content\":{\"connectorIds\":[]},\"type\":\"ConnectorPlacement.EquallySpacedRectSide\",\"uuid\":\"9b8fdd88-1c7e-48be-9cfb-0481a6997d70\"},{\"content\":{\"connectorIds\":[],\"side\":\"RIGHT\"},\"type\":\"ConnectorPlacement.EquallySpacedRectSide\",\"uuid\":\"09133262-ae09-4a08-942a-feb1f9e4bf66\"},{\"content\":{\"connectorIds\":[\"LConn1\"],\"side\":\"TOP\"},\"type\":\"ConnectorPlacement.EquallySpacedRectSide\",\"uuid\":\"b524eb7e-dd7a-431a-8842-4adf3b6cfedc\"}]},\"type\":\"ConnectorPlacement.EquallySpacedConnector\",\"uuid\":\"16ac0096-5732-49f8-94c0-648a6a453a34\"}],\"packageUris\":[\"http://schema.mathworks.com/mf0/Connector/19700101\"],\"version\":\"1.0\"}"
      mask Display: image('Sonar.png')
  Sonar2 : Subsystem
      settings: PortSchema="{\"entries\":[{\"content\":{\"sides\":[{\"content\":{\"connectorIds\":[]},\"type\":\"ConnectorPlacement.EquallySpacedRectSide\",\"uuid\":\"9b8fdd88-1c7e-48be-9cfb-0481a6997d70\"},{\"content\":{\"connectorIds\":[],\"side\":\"RIGHT\"},\"type\":\"ConnectorPlacement.EquallySpacedRectSide\",\"uuid\":\"09133262-ae09-4a08-942a-feb1f9e4bf66\"},{\"content\":{\"connectorIds\":[\"LConn1\"],\"side\":\"TOP\"},\"type\":\"ConnectorPlacement.EquallySpacedRectSide\",\"uuid\":\"b524eb7e-dd7a-431a-8842-4adf3b6cfedc\"}]},\"type\":\"ConnectorPlacement.EquallySpacedConnector\",\"uuid\":\"16ac0096-5732-49f8-94c0-648a6a453a34\"}],\"packageUris\":[\"http://schema.mathworks.com/mf0/Connector/19700101\"],\"version\":\"1.0\"}"
      mask Display: image('Sonar.png')
  StarboardPropMotor : Subsystem
      mask Display: image('PropMotor.png',[0,0.05,1,0.9])
  IMU : PMIOPort  Side=Left
  SP : PMIOPort  Port=2  Side=Left
  F : PMIOPort  Port=3  Side=Left
  PP : PMIOPort  Port=4  Side=Right
  connections:
  BatteryPack/LConn1 -- BottomStrip/LConn1 -- GPS/LConn1 -- StarboardPropMotor/RConn1 -- PortPropMotor/RConn1 -- Main_Hull/LConn1 -- DVL/LConn1 -- Sonar1/LConn1 -- ElectronicBoards/LConn2 -- Sonar2/LConn1 -- Camera/LConn1 -- ReferenceFrame/RConn1 -- Frame Alignment/RConn1
  IMU/RConn1 -- ElectronicBoards/LConn1
  Frame Alignment/LConn1 -- F/RConn1
  SP/RConn1 -- Frame Alignment/LConn2
  Frame Alignment/RConn2 -- PP/RConn1

== system AUV_ControlsPreliminary/AUV/Muiltibody/AUV Mechanics/AUVBody/SternHorThrusterTunnel ==
  ReferenceFrame : sm_lib/Frames and Transforms/Reference Frame
  SternHorThrusterMount : Subsystem
      mask Display: image('ThrusterMount.png')
  Stern_Horizontal_Thruster_Tunnel : Subsystem
      mask Display: image('HorizontalTunnel.png')
  T1 : sm_lib/Frames and Transforms/Rigid Transform  TranslationMethod=Cartesian  TranslationStandardOffset=0  TranslationLengthUnit=m  TranslationStandardAxis=+Z  TranslationCartesianOffset=smiData.RigidTransform(83).translation  TranslationROffset=0  TranslationROffsetUnits=m  TranslationZOffset=0  TranslationZOffsetUnits=m  TranslationThetaOffset=0  TranslationThetaOffsetUnits=deg  RotationMethod=ArbitraryAxis  RotationAngleUnits=rad  RotationStandardAxis=+Z  RotationAngle=smiData.RigidTransform(83).angle  RotationArbitraryAxis=smiData.RigidTransform(83).axis  FollAlignAxisA=+X  BaseAlignAxisA=+Y  FollAlignAxisB=+Y  BaseAlignAxisB=+Z  RotationSequenceAxes=FollowerAxes  RotationSequence=XYX  RotationSequenceAngles=[0 0 0]  RotationSequenceAnglesUnits=deg  RotationMatrix=[1 0 0; 0 1 0; 0 0 1]
  T2 : sm_lib/Frames and Transforms/Rigid Transform  TranslationMethod=Cartesian  TranslationStandardOffset=0  TranslationLengthUnit=m  TranslationStandardAxis=+Z  TranslationCartesianOffset=smiData.RigidTransform(92).translation  TranslationROffset=0  TranslationROffsetUnits=m  TranslationZOffset=0  TranslationZOffsetUnits=m  TranslationThetaOffset=0  TranslationThetaOffsetUnits=deg  RotationMethod=ArbitraryAxis  RotationAngleUnits=rad  RotationStandardAxis=+Z  RotationAngle=smiData.RigidTransform(92).angle  RotationArbitraryAxis=smiData.RigidTransform(92).axis  FollAlignAxisA=+X  BaseAlignAxisA=+Y  FollAlignAxisB=+Y  BaseAlignAxisB=+Z  RotationSequenceAxes=FollowerAxes  RotationSequence=XYX  RotationSequenceAngles=[0 0 0]  RotationSequenceAnglesUnits=deg  RotationMatrix=[1 0 0; 0 1 0; 0 0 1]
  T3 : sm_lib/Frames and Transforms/Rigid Transform  TranslationMethod=Cartesian  TranslationStandardOffset=0  TranslationLengthUnit=m  TranslationStandardAxis=+Z  TranslationCartesianOffset=smiData.RigidTransform(11).translation  TranslationROffset=0  TranslationROffsetUnits=m  TranslationZOffset=0  TranslationZOffsetUnits=m  TranslationThetaOffset=0  TranslationThetaOffsetUnits=deg  RotationMethod=ArbitraryAxis  RotationAngleUnits=rad  RotationStandardAxis=+Z  RotationAngle=smiData.RigidTransform(11).angle  RotationArbitraryAxis=smiData.RigidTransform(11).axis  FollAlignAxisA=+X  BaseAlignAxisA=+Y  FollAlignAxisB=+Y  BaseAlignAxisB=+Z  RotationSequenceAxes=FollowerAxes  RotationSequence=XYX  RotationSequenceAngles=[0 0 0]  RotationSequenceAnglesUnits=deg  RotationMatrix=[1 0 0; 0 1 0; 0 0 1]
  F : PMIOPort  Side=Left
  SHT : PMIOPort  Port=2  Side=Right
  connections:
  T2/LConn1 -- T3/LConn1 -- F/RConn1
  ReferenceFrame/RConn1 -- T1/LConn1 -- T2/RConn1 -- SternHorThrusterMount/LConn1
  Stern_Horizontal_Thruster_Tunnel/LConn1 -- T1/RConn1
  SHT/RConn1 -- T3/RConn1

== system AUV_ControlsPreliminary/AUV/Muiltibody/AUV Mechanics/AUVBody/SternHullCap ==
  Comms_Modem : Subsystem
      mask Display: image('Modem.png')
  ReferenceFrame : sm_lib/Frames and Transforms/Reference Frame
  Stern_Hull_Cap : Subsystem
      mask Display: image('SternHullCap.png')
  T1 : sm_lib/Frames and Transforms/Rigid Transform  TranslationMethod=Cartesian  TranslationStandardOffset=0  TranslationLengthUnit=m  TranslationStandardAxis=+Z  TranslationCartesianOffset=smiData.RigidTransform(41).translation  TranslationROffset=0  TranslationROffsetUnits=m  TranslationZOffset=0  TranslationZOffsetUnits=m  TranslationThetaOffset=0  TranslationThetaOffsetUnits=deg  RotationMethod=ArbitraryAxis  RotationAngleUnits=rad  RotationStandardAxis=+Z  RotationAngle=smiData.RigidTransform(41).angle  RotationArbitraryAxis=smiData.RigidTransform(41).axis  FollAlignAxisA=+X  BaseAlignAxisA=+Y  FollAlignAxisB=+Y  BaseAlignAxisB=+Z  RotationSequenceAxes=FollowerAxes  RotationSequence=XYX  RotationSequenceAngles=[0 0 0]  RotationSequenceAnglesUnits=deg  RotationMatrix=[1 0 0; 0 1 0; 0 0 1]
  T2 : sm_lib/Frames and Transforms/Rigid Transform  TranslationMethod=Cartesian  TranslationStandardOffset=0  TranslationLengthUnit=m  TranslationStandardAxis=+Z  TranslationCartesianOffset=smiData.RigidTransform(42).translation  TranslationROffset=0  TranslationROffsetUnits=m  TranslationZOffset=0  TranslationZOffsetUnits=m  TranslationThetaOffset=0  TranslationThetaOffsetUnits=deg  RotationMethod=ArbitraryAxis  RotationAngleUnits=rad  RotationStandardAxis=+Z  RotationAngle=smiData.RigidTransform(42).angle  RotationArbitraryAxis=smiData.RigidTransform(42).axis  FollAlignAxisA=+X  BaseAlignAxisA=+Y  FollAlignAxisB=+Y  BaseAlignAxisB=+Z  RotationSequenceAxes=FollowerAxes  RotationSequence=XYX  RotationSequenceAngles=[0 0 0]  RotationSequenceAnglesUnits=deg  RotationMatrix=[1 0 0; 0 1 0; 0 0 1]
  T3 : sm_lib/Frames and Transforms/Rigid Transform  TranslationMethod=Cartesian  TranslationStandardOffset=0  TranslationLengthUnit=m  TranslationStandardAxis=+Z  TranslationCartesianOffset=smiData.RigidTransform(43).translation  TranslationROffset=0  TranslationROffsetUnits=m  TranslationZOffset=0  TranslationZOffsetUnits=m  TranslationThetaOffset=0  TranslationThetaOffsetUnits=deg  RotationMethod=ArbitraryAxis  RotationAngleUnits=rad  RotationStandardAxis=+Z  RotationAngle=smiData.RigidTransform(43).angle  RotationArbitraryAxis=smiData.RigidTransform(43).axis  FollAlignAxisA=+X  BaseAlignAxisA=+Y  FollAlignAxisB=+Y  BaseAlignAxisB=+Z  RotationSequenceAxes=FollowerAxes  RotationSequence=XYX  RotationSequenceAngles=[0 0 0]  RotationSequenceAnglesUnits=deg  RotationMatrix=[1 0 0; 0 1 0; 0 0 1]
  T4 : sm_lib/Frames and Transforms/Rigid Transform  TranslationMethod=StandardAxis  TranslationStandardOffset=0.0135  TranslationLengthUnit=m  TranslationStandardAxis=+Y  TranslationCartesianOffset=[0 0 0]  TranslationROffset=0  TranslationROffsetUnits=m  TranslationZOffset=0  TranslationZOffsetUnits=m  TranslationThetaOffset=0  TranslationThetaOffsetUnits=deg  RotationMethod=None  RotationAngleUnits=deg  RotationStandardAxis=+Z  RotationAngle=0.0  RotationArbitraryAxis=[0 0 1]  FollAlignAxisA=+X  BaseAlignAxisA=+Y  FollAlignAxisB=+Y  BaseAlignAxisB=+Z  RotationSequenceAxes=FollowerAxes  RotationSequence=XYX  RotationSequenceAngles=[0 0 0]  RotationSequenceAnglesUnits=deg  RotationMatrix=[1 0 0; 0 1 0; 0 0 1]
  F : PMIOPort  Side=Left
  connections:
  T4/LConn1 -- T2/RConn1
  T3/LConn1 -- F/RConn1
  T2/LConn1 -- T3/RConn1 -- ReferenceFrame/RConn1 -- T1/LConn1
  Comms_Modem/LConn1 -- T4/RConn1
  Stern_Hull_Cap/LConn1 -- T1/RConn1

== system AUV_ControlsPreliminary/AUV/Muiltibody/AUV Mechanics/AUVBody/SternVerThrusterTunnel ==
  ReferenceFrame : sm_lib/Frames and Transforms/Reference Frame
  SternVerThrusterMount : Subsystem
      mask Display: image('ThrusterMount.png')
  Stern_Vertical_Thruster_Tunnel : Subsystem
      mask Display: image('VerticalTunnel.png')
  T1 : sm_lib/Frames and Transforms/Rigid Transform  TranslationMethod=Cartesian  TranslationStandardOffset=0  TranslationLengthUnit=m  TranslationStandardAxis=+Z  TranslationCartesianOffset=smiData.RigidTransform(93).translation  TranslationROffset=0  TranslationROffsetUnits=m  TranslationZOffset=0  TranslationZOffsetUnits=m  TranslationThetaOffset=0  TranslationThetaOffsetUnits=deg  RotationMethod=ArbitraryAxis  RotationAngleUnits=rad  RotationStandardAxis=+Z  RotationAngle=smiData.RigidTransform(93).angle  RotationArbitraryAxis=smiData.RigidTransform(93).axis  FollAlignAxisA=+X  BaseAlignAxisA=+Y  FollAlignAxisB=+Y  BaseAlignAxisB=+Z  RotationSequenceAxes=FollowerAxes  RotationSequence=XYX  RotationSequenceAngles=[0 0 0]  RotationSequenceAnglesUnits=deg  RotationMatrix=[1 0 0; 0 1 0; 0 0 1]
  T2 : sm_lib/Frames and Transforms/Rigid Transform  TranslationMethod=Cartesian  TranslationStandardOffset=0  TranslationLengthUnit=m  TranslationStandardAxis=+Z  TranslationCartesianOffset=smiData.RigidTransform(102).translation  TranslationROffset=0  TranslationROffsetUnits=m  TranslationZOffset=0  TranslationZOffsetUnits=m  TranslationThetaOffset=0  TranslationThetaOffsetUnits=deg  RotationMethod=ArbitraryAxis  RotationAngleUnits=rad  RotationStandardAxis=+Z  RotationAngle=smiData.RigidTransform(102).angle  RotationArbitraryAxis=smiData.RigidTransform(102).axis  FollAlignAxisA=+X  BaseAlignAxisA=+Y  FollAlignAxisB=+Y  BaseAlignAxisB=+Z  RotationSequenceAxes=FollowerAxes  RotationSequence=XYX  RotationSequenceAngles=[0 0 0]  RotationSequenceAnglesUnits=deg  RotationMatrix=[1 0 0; 0 1 0; 0 0 1]
  T3 : sm_lib/Frames and Transforms/Rigid Transform  TranslationMethod=Cartesian  TranslationStandardOffset=0  TranslationLengthUnit=m  TranslationStandardAxis=+Z  TranslationCartesianOffset=smiData.RigidTransform(5).translation  TranslationROffset=0  TranslationROffsetUnits=m  TranslationZOffset=0  TranslationZOffsetUnits=m  TranslationThetaOffset=0  TranslationThetaOffsetUnits=deg  RotationMethod=ArbitraryAxis  RotationAngleUnits=rad  RotationStandardAxis=+Z  RotationAngle=smiData.RigidTransform(5).angle  RotationArbitraryAxis=smiData.RigidTransform(5).axis  FollAlignAxisA=+X  BaseAlignAxisA=+Y  FollAlignAxisB=+Y  BaseAlignAxisB=+Z  RotationSequenceAxes=FollowerAxes  RotationSequence=XYX  RotationSequenceAngles=[0 0 0]  RotationSequenceAnglesUnits=deg  RotationMatrix=[1 0 0; 0 1 0; 0 0 1]
  F : PMIOPort  Side=Left
  SVT : PMIOPort  Port=2  Side=Right
  connections:
  T2/LConn1 -- T3/LConn1 -- F/RConn1
  ReferenceFrame/RConn1 -- T1/LConn1 -- T2/RConn1 -- SternVerThrusterMount/LConn1
  Stern_Vertical_Thruster_Tunnel/LConn1 -- T1/RConn1
  SVT/RConn1 -- T3/RConn1
